simulink model "ident_model"  (R2021a)
settings: Solver=VariableStepAuto  StartTime=0.0  StopTime=1000  RelTol=1e-3
settings Model: Creator=marti  LastModifiedBy=marti

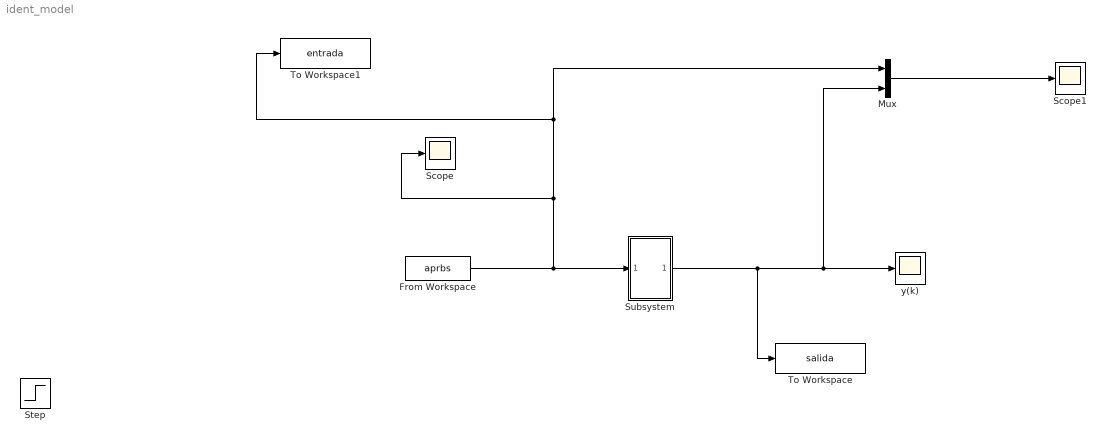
== system ident_model ==
  From Workspace : FromWorkspace  VariableName=aprbs  SampleTime=0.1
  Mux : Mux  Inputs=2
  Scope : Scope
  Scope1 : Scope
  Step : Step  SampleTime=0
  Subsystem : Subsystem
  To Workspace : ToWorkspace  VariableName=salida  SampleTime=-1
  To Workspace1 : ToWorkspace  VariableName=entrada  SampleTime=-1
  y(k) : Scope
  wires:
  From Workspace/1 -> Mux/1, To Workspace1/1, Scope/1, Subsystem/1(In1)
  Subsystem/1(Out1) -> To Workspace/1, Mux/2, y(k)/1
  Mux/1 -> Scope1/1

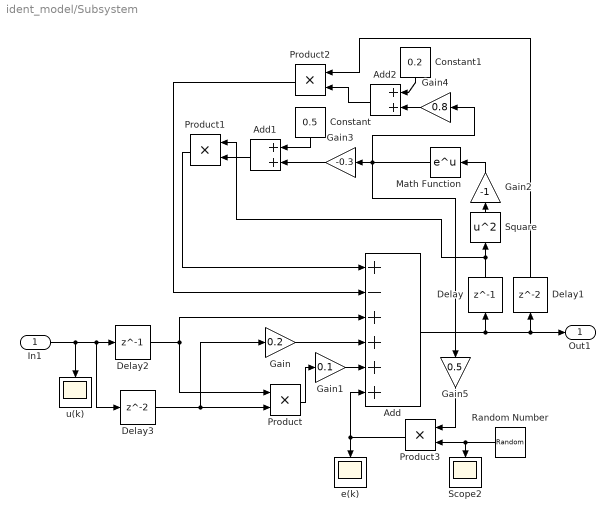
== system ident_model/Subsystem ==
  In1 : Inport
  Add : Sum  Inputs=+-++++
  Add1 : Sum
  Add2 : Sum
  Constant : Constant  Value=0.5
  Constant1 : Constant  Value=0.2
  Delay : Delay  DelayLength=1  InitialCondition=0
  Delay1 : Delay
  Delay2 : Delay  DelayLength=1  InitialCondition=0
  Delay3 : Delay
  Gain : Gain  Gain=0.2
  Gain1 : Gain  Gain=0.1
  Gain2 : Gain  Gain=-1
  Gain3 : Gain  Gain=-0.3
  Gain4 : Gain  Gain=0.8
  Gain5 : Gain  Gain=0.5
  Math Function : Math  SaturateOnIntegerOverflow=on
  Product{,1..3} (4 alike) : Product
  Random Number : RandomNumber  SampleTime=0.1
  Scope2 : Scope
  Square : Math  Operator=square  SaturateOnIntegerOverflow=on
  e(k) : Scope
  u(k) : Scope
  Out1 : Outport
  wires:
  Delay3/1 -> Product/2, Gain/1
  Gain1/1 -> Add/5
  Delay2/1 -> Product/1, Add/3
  Delay/1 -> Product1/1, Square/1
  Gain/1 -> Add/4
  Math Function/1 -> Gain4/1, Gain3/1, Gain5/1
  Square/1 -> Gain2/1
  In1/1 -> u(k)/1, Delay3/1, Delay2/1
  Random Number/1 -> Product3/2, Scope2/1
  Constant1/1 -> Add2/1
  Add/1 -> Delay/1, Out1/1, Delay1/1
  Delay1/1 -> Product2/1
  Gain5/1 -> Product3/1
  Add1/1 -> Product1/2
  Product3/1 -> Add/6, e(k)/1
  Add2/1 -> Product2/2
  Constant/1 -> Add1/1
  Product2/1 -> Add/2
  Gain3/1 -> Add1/2
  Gain4/1 -> Add2/2
  Product1/1 -> Add/1
  Gain2/1 -> Math Function/1
  Product/1 -> Gain1/1
